simulink model "Control_PF_v2013a"  (Simulink 8.1)
settings: Solver=ode45  SolverMode=SingleTasking  StartTime=0.0  StopTime=120  RelTol=1e-3
values from neighbouring files (symbols this model uses):
  b = 0.0425    [parte1_eje7_Control_PF_datos.m]
  Ki = 0.09    [parte1_eje7_Control_PF_datos.m]
  Kps = 100    [parte1_eje7_Control_PF_datos.m]
  R = rlocus(G,K)    [parte1_eje11_lugarderaices.m]    (also in parte1_eje1_circuitoRC.m = 10; parte1_eje2_circuitoRLC.m = 10000; parte1_eje4_SScircuitoRLC.m = 100; parte1_eje5_ft_circuitoRLC.m = 100)
  Tps = 20    [parte1_eje7_Control_PF_datos.m]
  Tt = 0.5    [parte1_eje7_Control_PF_datos.m]
undefined symbols (not defined in the file or in its folder): Tsg
settings Model: Creator=N. Quintanilla  LastModifiedBy=cjuar  CovMetricSettings=dwe  CovHtmlReporting=off  covSaveCumulativeToWorkspaceVar=off  CovSaveSingleToWorkspaceVar=off  CovExternalEMLEnable=on
settings DataIOCC: LimitDataPoints=off  SaveFormat=StructureWithTime  SignalLoggingSaveFormat=Dataset
settings OptimizationCC: ExpressionDepthLimit=128
settings DebuggingCC: UnderspecifiedInitializationDetection=Simplified  MergeDetectMultiDrivingBlocksExec=error  SolverPrmCheckMsg=none  FcnCallInpInsideContextMsg=EnableAllAsError  FrameProcessingCompatibilityMsg=error  StateNameClashWarn=none  SFUnexpectedBacktrackingDiag=error  SFNoUnconditionalDefaultTransitionDiag=error
settings HardwareCC: ProdBitPerPointer=64  ProdLargestAtomicFloat=Float  ProdIntDivRoundTo=Zero  ProdEndianess=LittleEndian  ProdHWDeviceType=Specified
settings ModelReferenceCC: PropagateSignalLabelsOutOfModel=on
settings GRTTargetCC: CodeReplacementLibrary=C99 (ISO)  GeneratePreprocessorConditionals=Use local settings  CombineOutputUpdateFcns=on  GRTInterface=off

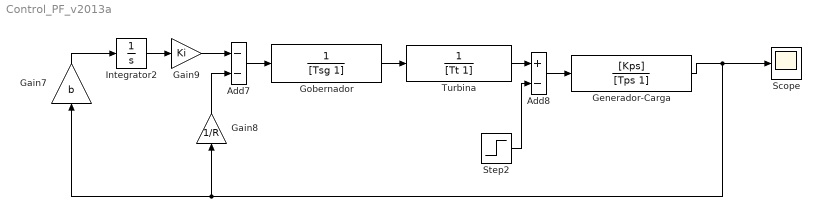
== system Control_PF_v2013a ==
  " Generador-Carga" : TransferFcn  Numerator=[Kps]  Denominator=[Tps 1]
  Add7 : Sum  Inputs=--
  Add8 : Sum  Inputs=+-
  Gain7 : Gain  Gain=b
  Gain8 : Gain  Gain=1/R
  Gain9 : Gain  Gain=Ki
  Gobernador : TransferFcn  Denominator=[Tsg 1]
  Integrator2 : Integrator
  Scope : Scope
      settings: TimeRange=auto  MaxDataPoints=5000  SaveToWorkspace=off  YMin=-0.05111  YMax=0.0057  SampleTime=-1
  Step2 : Step  Time=0  After=.01  SampleTime=0
  "Turbina " : TransferFcn  Denominator=[Tt 1]
  wires:
  "Turbina "/1 -> Add8/1
  Step2/1 -> Add8/2
  Gain9/1 -> Add7/1
  Add8/1 -> " Generador-Carga"/1
  Gain7/1 -> Integrator2/1
  Integrator2/1 -> Gain9/1
  Gain8/1 -> Add7/2
  " Generador-Carga"/1 -> Gain8/1, Gain7/1, Scope/1
  Add7/1 -> Gobernador/1
  Gobernador/1 -> "Turbina "/1
